simulink model "vehicle_cruise_control"  (R2025a)
settings: Solver=VariableStepAuto  StartTime=0.0  StopTime=1000  RelTol=1e-3
libraries: slpidlib x1
settings Model: Creator=nima9  LastModifiedBy=nima9

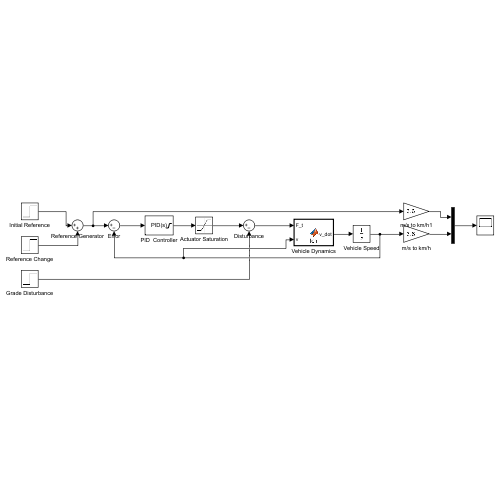
[thumbnail: Simulink's stored preview of the top-level diagram]
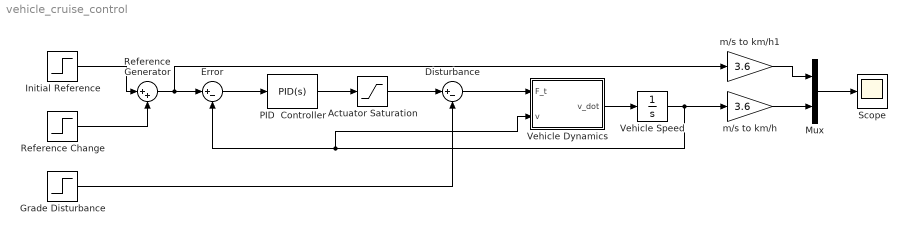
== system vehicle_cruise_control ==
  Actuator Saturation : Saturate  UpperLimit=6000  LowerLimit=0
  Disturbance : Sum  Inputs=|+-
  Error : Sum  Inputs=|+-
  Grade Disturbance : Step  Time=600  After=500  SampleTime=0
  Initial Reference : Step  Time=0  After=16.6667  SampleTime=0
  Mux : Mux  Inputs=2
  PID  Controller : slpidlib/PID Controller  Controller=PID  Form=Parallel  TimeDomain=Continuous-time  UseExternalTs=off  SampleTime=-1  IntegratorMethod=Forward Euler  FilterMethod=Forward Euler  ControllerParametersSource=internal  P=100  I=1  UseKiTs=off  D=10  UseExternalDerivativeSource=off  N=100  UseFilter=on  TunerSelectOption=Transfer Function Based (PID Tuner App)  InitialConditionSource=internal  InitialConditionForIntegrator=0  InitialConditionForFilter=0  DifferentiatorICPrevScaledInput=0  ExternalReset=none  TrackingMode=off  Kt=1  LimitOutput=on  SatLimitsSource=internal  UpperSaturationLimit=inf  LowerSaturationLimit=-inf  LinearizeAsGain=on  AntiWindupMode=back-calculation  Kb=1  LimitIntegrator=off  UpperIntegratorSaturationLimit=inf  LowerIntegratorSaturationLimit=-inf  POutMin=[]  POutMax=[]  IOutMin=[]  IOutMax=[]  DOutMin=[]  DOutMax=[]  NOutMin=[]  NOutMax=[]  SumOutMin=[]  SumOutMax=[]  SaturationOutMin=[]  SaturationOutMax=[]  PParamMin=[]  PParamMax=[]  IParamMin=[]  IParamMax=[]  DParamMin=[]  DParamMax=[]  NParamMin=[]  NParamMax=[]  KbParamMin=[]  KbParamMax=[]  KtParamMin=[]  KtParamMax=[]  KbOutMin=[]  KbOutMax=[]  KtOutMin=[]  KtOutMax=[]  IntegratorOutMin=[]  IntegratorOutMax=[]  FilterOutMin=[]  FilterOutMax=[]  SumI1OutMin=[]  SumI1OutMax=[]  SumI2OutMin=[]  SumI2OutMax=[]  SumI3OutMin=[]  SumI3OutMax=[]  SumI4OutMin=[]  SumI4OutMax=[]  SumDOutMin=[]  SumDOutMax=[]  DifferentiatorOutMin=[]  DifferentiatorOutMax=[]  FilterDiffOutCoefMin=[]  FilterDiffOutCoefMax=[]  ReciprocalOutMin=[]  ReciprocalOutMax=[]  SumDenOutMin=[]  SumDenOutMax=[]  SumNumOutMin=[]  SumNumOutMax=[]  DivideOutMin=[]  DivideOutMax=[]  UdiffTsProdOutMin=[]  UdiffTsProdOutMax=[]  NTsProdOutMin=[]  NTsProdOutMax=[]  UintegralTsProdOutMin=[]  UintegralTsProdOutMax=[]  UngainTsProdOutMin=[]  UngainTsProdOutMax=[]  ClampingZeroOutDataTypeStr=Inherit: Inherit via back propagation  ClampingZeroOutMin=[]  ClampingZeroOutMax=[]  FilterDenConstantOutDataTypeStr=Inherit: Inherit via back propagation  FilterDenConstantOutMin=[]  FilterDenConstantOutMax=[]  PCopyOutDataTypeStr=Inherit: Inherit via back propagation  PCopyOutMin=[]  PCopyOutMax=[]  NCopyOutDataTypeStr=Inherit: Inherit via back propagation  NCopyOutMin=[]  NCopyOutMax=[]  IntegratorContinuousStateAttributes=''  IntegratorStateMustResolveToSignalObject=off  IntegratorRTWStateStorageClass=Auto  FilterContinuousStateAttributes=''  FilterStateMustResolveToSignalObject=off  FilterRTWStateStorageClass=Auto  ParallelPVariant=InternalParameters  IdealPVariant=Disabled  IVariant=InternalParameters  DVariant=InternalParameters  IntegratorVariant=Continuous  SatVariant=Enabled  AWVariant=BackCalculation  PCopyVariant=Disabled  TRVariant=Disabled  FdbkBlocksVariant=Forward  IdealPFdbkVariant=Disabled  SatFdbkVariant=Disabled  DerivativeFilterVariant=ContFilter  NVariant=InternalParameters  NCopyVariant=Disabled  FilterICVariant=InternalICsFilter  IntegratorICVariant=InternalICs  ExternalResetVariant=Disabled  TRSumVariant=Passthrough  SumFdbkVariant=Disabled  SumVariant=Sum_PID  TsampFilterVariant=InternalTs  TsampNgainVariant=Passthrough  TsampIntegralVariant=Disabled_SignalSpec  ExternalSaturationOutDataTypeStr=Inherit: Same as second input  DerivativeSourceVariant=ErrorSignal  PreIntVariant=InternalPreInt
  Reference Change : Step  Time=400  After=11.1111  SampleTime=0
  Reference Generator : Sum  Inputs=|++
  Scope : Scope
      settings: ActiveDisplayYMinimum=-11.014155347117054  ActiveDisplayYMaximum=226.0074513070727
  Vehicle Dynamics : MATLAB Function  TreatAsAtomicUnit=on
  Vehicle Speed : Integrator
  m/s to km/h : Gain  Gain=3.6
  m/s to km/h1 : Gain  Gain=3.6
  wires:
  Initial Reference/1 -> Reference Generator/1
  Error/1 -> PID  Controller/1
  Vehicle Dynamics/1(v_dot) -> Vehicle Speed/1
  Vehicle Speed/1 -> m/s to km/h/1, Vehicle Dynamics/2(v), Error/2
  Reference Change/1 -> Reference Generator/2
  Reference Generator/1 -> m/s to km/h1/1, Error/1
  Disturbance/1 -> Vehicle Dynamics/1(F_t)
  Actuator Saturation/1 -> Disturbance/1
  PID  Controller/1 -> Actuator Saturation/1
  m/s to km/h/1 -> Mux/2
  m/s to km/h1/1 -> Mux/1
  Mux/1 -> Scope/1
  Grade Disturbance/1 -> Disturbance/2

== matlab function vehicle_cruise_control/Vehicle Dynamics ==
  data: F_t input; v_dot output; v input
function v_dot = fcn(F_t, v)

rho = 1.225;
Cd = 0.30;
A = 2.20;
Crr = 0.01;
m = 1500;
g = 9.81;

F_drag = 0.5 * rho * Cd * A * v^2;
F_rolling = Crr * m * g;

F_resistance = F_drag + F_rolling;

v_dot = (F_t - F_resistance) / m;

end
